simulink model "r2017bSingleARDroneCtrl"  (R2017b)
settings: Solver=FixedStepAuto  StartTime=0.0  StopTime=inf  FixedStep=sampleTime  RelTol=1e-3  EnableMultiTasking=on
values from neighbouring files (symbols this model uses):
  k = 1.0    (= 1)    [start.m]
  k_d_xy = 0.9    [start.m]
  k_d_z = 0.3    [start.m]
  k_l = 5    [start.m]
  k_p_xy = 0.6    [start.m]
  k_p_yaw = 0.5    [start.m]
  k_p_z = 0.6    [start.m]
  k_sign = -1    [start.m]
  limit_cmd_xy = 1    [start.m]
  r_a = 3    [start.m]
  r_M = 2    [start.m]
  r_o = 0.5    [start.m]
  r_s = 0.001    [start.m]
  waypoints = [1,1,1.2,0,0,0,0]'    [start.m]
undefined symbols (not defined in the file or in its folder): Angular, Linear
libraries: robotlib x5
settings Model: Creator=exbot  LastModifiedBy=gzl20
settings DataIOCC: LimitDataPoints=on
settings OptimizationCC: MaxStackSize=64
settings DebuggingCC: ParameterTunabilityLossMsg=error  AllowSymbolicDim=off  SFUnexpectedBacktrackingDiag=warning  SFNoUnconditionalDefaultTransitionDiag=warning  SFExecutionAtInitializationDiag=none
settings HardwareCC: ProdBitPerPointer=32  ProdBitPerSizeT=32  ProdBitPerPtrDiffT=32  ProdLargestAtomicFloat=None  ProdIntDivRoundTo=Undefined  ProdEndianess=Unspecified  ProdWordSize=32  ProdHWDeviceType=Generic->Unspecified (assume 32-bit Generic)
settings ModelReferenceCC: PropagateSignalLabelsOutOfModel=off
settings SFSimCC: MATLABDynamicMemAlloc=off
settings RTWCC: SystemTargetFile=ert.tlc  HardwareBoard=Robot Operating System (ROS)  TemplateMakefile=ert_default_tmf  Toolchain=Catkin  TargetLang=C++
settings CodeAppCC: ForceParamTrailComments=on  IgnoreCustomStorageClasses=off  OperatorAnnotations=on  SimulinkDataObjDesc=on  SFDataObjDesc=on  MATLABFcnDesc=on  InsertBlockDesc=on  StateflowObjectComments=on  MATLABSourceComments=on
settings ERTTargetCC: MultiwordLength=2048  SupportContinuousTime=on
settings ConfigComp: CovMetricSettings=dw  CovHtmlReporting=on  CovSaveCumulativeToWorkspaceVar=on  CovSaveSingleToWorkspaceVar=on  CovExternalEMLEnable=off

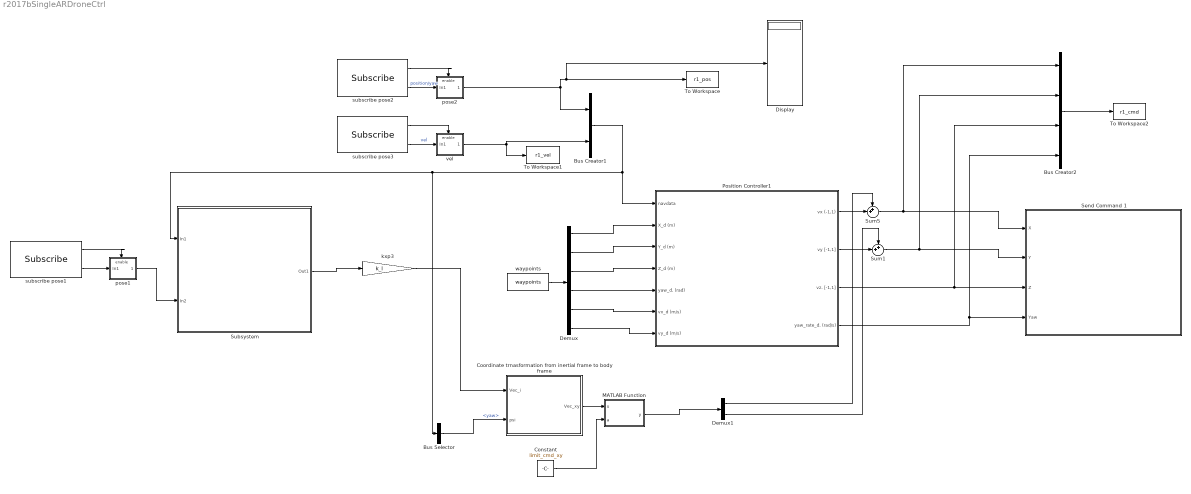
== system r2017bSingleARDroneCtrl ==
  Bus Creator1 : BusCreator  Inputs=2
  Bus Creator2 : BusCreator  Inputs=4
  Bus Selector : BusSelector  OutputSignals=signal1.yaw
  Constant : Constant  Value=limit_cmd_xy
  "Coordinate trnasformation from inertial frame to body frame " : MATLAB Function  TreatAsAtomicUnit=on
  Demux : Demux  Outputs=6
  Demux1 : Demux  Outputs=2
  Display : Display
  MATLAB Function : MATLAB Function  TreatAsAtomicUnit=on
  Position Controller1 : Subsystem  AncestorBlock=ARBlocks/Baseline Controller
  Send Command 1 : Subsystem
  Subsystem : Subsystem
  Sum1 : Sum  Inputs=++|
  Sum5 : Sum  Inputs=++|
  To Workspace : ToWorkspace  VariableName=r1_pos  SaveFormat=Timeseries  SampleTime=-1
  To Workspace1 : ToWorkspace  VariableName=r1_vel  SaveFormat=Timeseries  SampleTime=-1
  To Workspace2 : ToWorkspace  VariableName=r1_cmd  SaveFormat=Timeseries  SampleTime=-1
  kxp3 : Gain  Gain=k_l
  pose1 : Subsystem
  pose2 : Subsystem
  subscribe pose1 : robotlib/Subscribe  SourceLibraryInfo=This block requires Robotics System Toolbox  topicSource=Specify your own  topic=/Obstacle/position  messageType=geometry_msgs/Point  sampleTime=-1  messageQueueLength=1
      settings: SourceProductBaseCode=RO
  subscribe pose2 : robotlib/Subscribe  SourceLibraryInfo=This block requires Robotics System Toolbox  topicSource=Select from ROS network  topic=/Robot_1/pose  messageType=geometry_msgs/PoseStamped  sampleTime=-1  messageQueueLength=1
      settings: SourceProductBaseCode=RO
  subscribe pose3 : robotlib/Subscribe  SourceLibraryInfo=This block requires Robotics System Toolbox  topicSource=Select from ROS network  topic=/Robot_1/vel  messageType=geometry_msgs/PointStamped  sampleTime=-1  messageQueueLength=1
      settings: SourceProductBaseCode=RO
  vel : Subsystem
  waypoints : Constant  Value=waypoints  VectorParams1D=off
  wires:
  Position Controller1/3(vz. [-1,1]) -> Bus Creator2/3, Send Command 1/3(Z)
  Position Controller1/4(yaw_rate_d. (rad/s)) -> Bus Creator2/4, Send Command 1/4(Yaw)
  Bus Creator2/1 -> To Workspace2/1
  pose2/1(Out1) -> Bus Creator1/1, Display/1, To Workspace/1
  vel/1(Out1) -> Bus Creator1/2, To Workspace1/1
  Bus Creator1/1 -> Bus Selector/1, Subsystem/1(In1), Position Controller1/1(navdata)
  subscribe pose2/2 -> pose2/1(In1)  "position/yaw"
  subscribe pose2/1 -> pose2/Enable
  subscribe pose3/2 -> vel/1(In1)  "vel"
  subscribe pose3/1 -> vel/Enable
  subscribe pose1/2 -> pose1/1(In1)
  subscribe pose1/1 -> pose1/Enable
  pose1/1(Out1) -> Subsystem/2(In2)
  Subsystem/1(Out1) -> kxp3/1
  waypoints/1 -> Demux/1
  Demux/1 -> Position Controller1/2(X_d (m))
  Demux/2 -> Position Controller1/3(Y_d (m))
  Demux/3 -> Position Controller1/4(Z_d (m))
  Demux/4 -> Position Controller1/5(yaw_d. (rad))
  Demux/5 -> Position Controller1/6(vx_d (m/s))
  Demux/6 -> Position Controller1/7(vy_d (m/s))
  kxp3/1 -> "Coordinate trnasformation from inertial frame to body frame "/1(Vec_i)
  Position Controller1/1(vx (-1,1)) -> Sum5/2
  Sum5/1 -> Bus Creator2/1, Send Command 1/1(X)
  Sum1/1 -> Bus Creator2/2, Send Command 1/2(Y)
  Position Controller1/2(vy [-1,1]) -> Sum1/2
  Constant/1 -> MATLAB Function/2(a)
  "Coordinate trnasformation from inertial frame to body frame "/1(Vec_xy) -> MATLAB Function/1(u)
  Bus Selector/1 -> "Coordinate trnasformation from inertial frame to body frame "/2(psi)  "<yaw>"
  MATLAB Function/1(y) -> Demux1/1
  Demux1/1 -> Sum5/1
  Demux1/2 -> Sum1/1

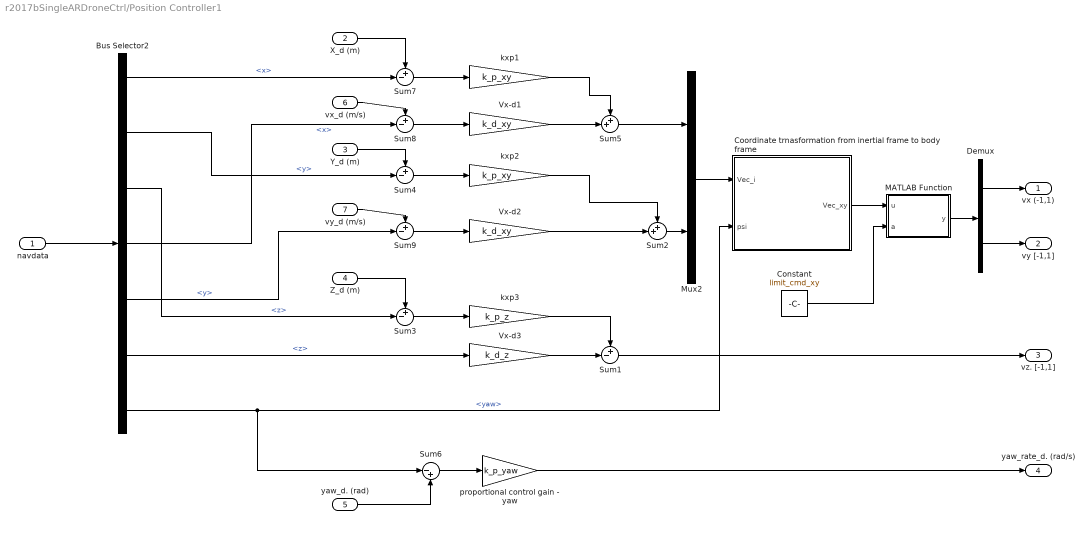
== system r2017bSingleARDroneCtrl/Position Controller1 ==
  navdata : Inport
  X_d (m) : Inport  Port=2
  Y_d (m) : Inport  Port=3
  Z_d (m) : Inport  Port=4
  yaw_d. (rad) : Inport  Port=5
  vx_d (m/s) : Inport  Port=6
  vy_d (m/s) : Inport  Port=7
  Bus Selector2 : BusSelector  OutputSignals=signal1.x,signal1.y,signal1.z,signal2.x,signal2.y,signal2.z,signal1.yaw
  Constant : Constant  Value=limit_cmd_xy
  "Coordinate trnasformation from inertial frame to body frame " : MATLAB Function  TreatAsAtomicUnit=on
  Demux : Demux  Outputs=2
  MATLAB Function : MATLAB Function  TreatAsAtomicUnit=on
  Mux2 : Mux  Inputs=2
  Sum{1,3..4,7..9} (6 alike) : Sum  Inputs=+-|
  Sum2 : Sum  Inputs=++|
  Sum5 : Sum  Inputs=++|
  Sum6 : Sum  Inputs=|-+
  Vx-d1 : Gain  Gain=k_d_xy
  Vx-d2 : Gain  Gain=k_d_xy
  Vx-d3 : Gain  Gain=k_d_z
  kxp1 : Gain  Gain=k_p_xy
  kxp2 : Gain  Gain=k_p_xy
  kxp3 : Gain  Gain=k_p_z
  proportional control gain - yaw : Gain  Gain=k_p_yaw
  vx (-1,1) : Outport
  vy [-1,1] : Outport  Port=2
  vz. [-1,1] : Outport  Port=3
  yaw_rate_d. (rad/s) : Outport  Port=4
  wires:
  MATLAB Function/1(y) -> Demux/1
  Demux/1 -> vx (-1,1)/1
  Demux/2 -> vy [-1,1]/1
  Constant/1 -> MATLAB Function/2(a)
  Mux2/1 -> "Coordinate trnasformation from inertial frame to body frame "/1(Vec_i)
  Sum7/1 -> kxp1/1
  kxp1/1 -> Sum5/1
  Vx-d1/1 -> Sum5/2
  X_d (m)/1 -> Sum7/1
  Sum4/1 -> kxp2/1
  kxp2/1 -> Sum2/1
  Vx-d2/1 -> Sum2/2
  Y_d (m)/1 -> Sum4/1
  Sum3/1 -> kxp3/1
  kxp3/1 -> Sum1/1
  Vx-d3/1 -> Sum1/2
  Z_d (m)/1 -> Sum3/1
  Bus Selector2/1 -> Sum7/2  "<x>"
  Bus Selector2/2 -> Sum4/2  "<y>"
  Bus Selector2/3 -> Sum3/2  "<z>"
  Bus Selector2/6 -> Vx-d3/1  "<z>"
  Bus Selector2/7 -> Sum6/1, "Coordinate trnasformation from inertial frame to body frame "/2(psi)  "<yaw>"
  Sum6/1 -> proportional control gain - yaw/1
  proportional control gain - yaw/1 -> yaw_rate_d. (rad/s)/1
  yaw_d. (rad)/1 -> Sum6/2
  navdata/1 -> Bus Selector2/1
  Sum5/1 -> Mux2/1
  Sum2/1 -> Mux2/2
  Sum1/1 -> vz. [-1,1]/1
  "Coordinate trnasformation from inertial frame to body frame "/1(Vec_xy) -> MATLAB Function/1(u)
  Bus Selector2/4 -> Sum8/2  "<x>"
  vx_d (m/s)/1 -> Sum8/1
  Sum8/1 -> Vx-d1/1
  Sum9/1 -> Vx-d2/1
  Bus Selector2/5 -> Sum9/2  "<y>"
  vy_d (m/s)/1 -> Sum9/1

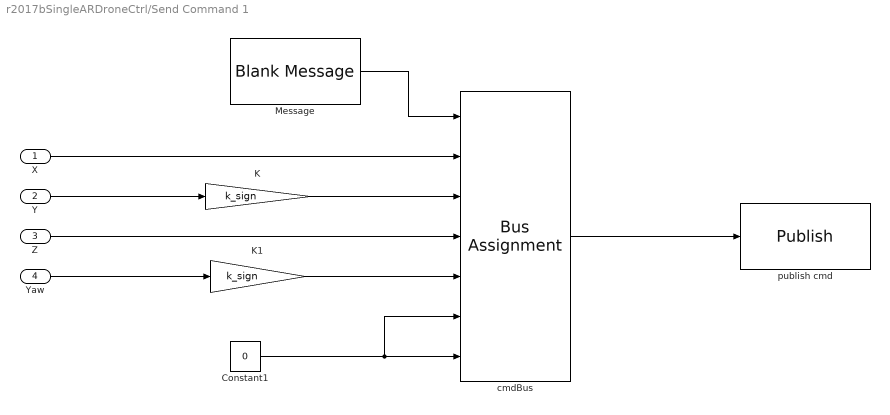
== system r2017bSingleARDroneCtrl/Send Command 1 ==
  X : Inport
  Y : Inport  Port=2
  Z : Inport  Port=3
  Yaw : Inport  Port=4
  " Message" : robotlib/Blank Message  SourceLibraryInfo=This block requires Robotics System Toolbox  messageType=geometry_msgs/Twist  SampleTime=inf
      settings: SourceProductBaseCode=RO
  Constant1 : Constant  Value=0
  K : Gain  Gain=k_sign
  K1 : Gain  Gain=k_sign
  cmdBus : BusAssignment  AssignedSignals=Linear.X,Linear.Y,Linear.Z,Angular.Z,Angular.X,Angular.Y
  publish cmd : robotlib/Publish  SourceLibraryInfo=This block requires Robotics System Toolbox  topicSource=Select from ROS network  topic=/bebop1/cmd_vel  messageType=geometry_msgs/Twist  messageQueueLength=1
      settings: SourceProductBaseCode=RO
  wires:
  cmdBus/1 -> publish cmd/1
  Constant1/1 -> cmdBus/6, cmdBus/7
  K/1 -> cmdBus/3
  K1/1 -> cmdBus/5
  " Message"/1 -> cmdBus/1
  X/1 -> cmdBus/2
  Y/1 -> K/1
  Z/1 -> cmdBus/4
  Yaw/1 -> K1/1

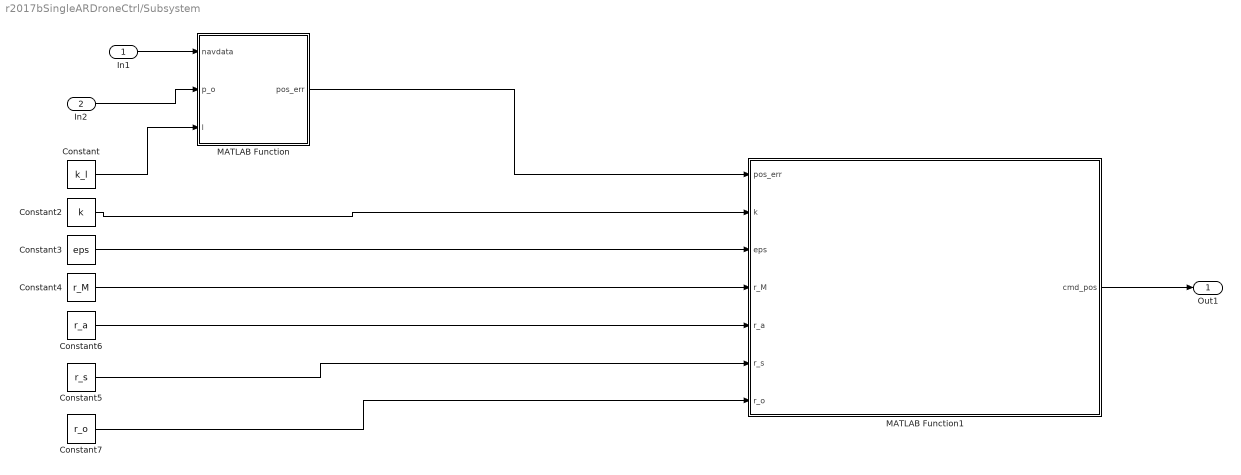
== system r2017bSingleARDroneCtrl/Subsystem ==
  In1 : Inport
  In2 : Inport  Port=2
  Constant : Constant  Value=k_l
  Constant2 : Constant  Value=k
  Constant3 : Constant  Value=eps
  Constant4 : Constant  Value=r_M
  Constant5 : Constant  Value=r_s
  Constant6 : Constant  Value=r_a
  Constant7 : Constant  Value=r_o
  MATLAB Function : MATLAB Function  TreatAsAtomicUnit=on
  MATLAB Function1 : MATLAB Function  TreatAsAtomicUnit=on
  Out1 : Outport
  wires:
  In1/1 -> MATLAB Function/1(navdata)
  In2/1 -> MATLAB Function/2(p_o)
  MATLAB Function/1(pos_err) -> MATLAB Function1/1(pos_err)
  Constant/1 -> MATLAB Function/3(l)
  Constant2/1 -> MATLAB Function1/2(k)
  Constant3/1 -> MATLAB Function1/3(eps)
  Constant4/1 -> MATLAB Function1/4(r_M)
  Constant6/1 -> MATLAB Function1/5(r_a)
  Constant5/1 -> MATLAB Function1/6(r_s)
  Constant7/1 -> MATLAB Function1/7(r_o)
  MATLAB Function1/1(cmd_pos) -> Out1/1

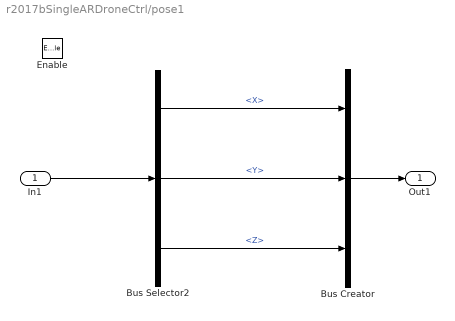
== system r2017bSingleARDroneCtrl/pose1 ==
  In1 : Inport
  Enable : EnablePort
  Bus Creator : BusCreator  Inputs=3
  Bus Selector2 : BusSelector  OutputSignals=X,Y,Z
  Out1 : Outport
  wires:
  Bus Creator/1 -> Out1/1
  In1/1 -> Bus Selector2/1
  Bus Selector2/1 -> Bus Creator/1  "<X>"
  Bus Selector2/2 -> Bus Creator/2  "<Y>"
  Bus Selector2/3 -> Bus Creator/3  "<Z>"

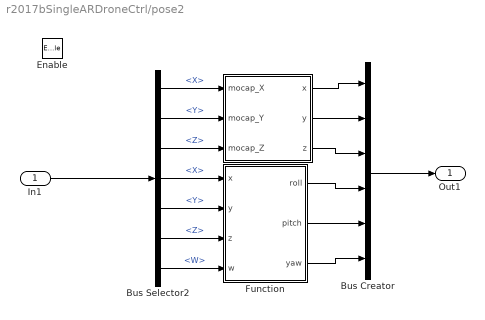
== system r2017bSingleARDroneCtrl/pose2 ==
  In1 : Inport
  Enable : EnablePort
  " " : MATLAB Function  TreatAsAtomicUnit=on
  " Function" : MATLAB Function  TreatAsAtomicUnit=on
  Bus Creator : BusCreator  Inputs=6
  Bus Selector2 : BusSelector  OutputSignals=Pose.Position.X,Pose.Position.Y,Pose.Position.Z,Pose.Orientation.X,Pose.Orientation.Y,Pose.Orientation.Z,Pose.Orientation.W
  Out1 : Outport
  wires:
  Bus Creator/1 -> Out1/1
  In1/1 -> Bus Selector2/1
  " Function"/1(roll) -> Bus Creator/4
  " Function"/2(pitch) -> Bus Creator/5
  " Function"/3(yaw) -> Bus Creator/6
  Bus Selector2/4 -> " Function"/1(x)  "<X>"
  Bus Selector2/5 -> " Function"/2(y)  "<Y>"
  Bus Selector2/6 -> " Function"/3(z)  "<Z>"
  Bus Selector2/7 -> " Function"/4(w)  "<W>"
  Bus Selector2/1 -> " "/1(mocap_X)  "<X>"
  Bus Selector2/2 -> " "/2(mocap_Y)  "<Y>"
  Bus Selector2/3 -> " "/3(mocap_Z)  "<Z>"
  " "/1(x) -> Bus Creator/1
  " "/2(y) -> Bus Creator/2
  " "/3(z) -> Bus Creator/3

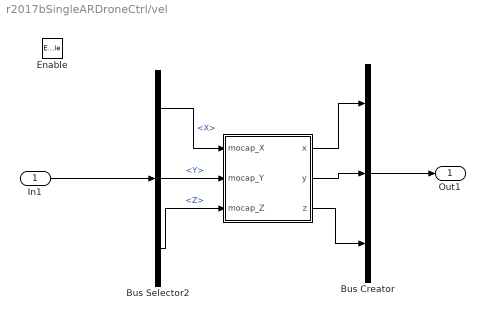
== system r2017bSingleARDroneCtrl/vel ==
  In1 : Inport
  Enable : EnablePort
  " " : MATLAB Function  TreatAsAtomicUnit=on
  Bus Creator : BusCreator  Inputs=3
  Bus Selector2 : BusSelector  OutputSignals=Point.X,Point.Y,Point.Z
  Out1 : Outport
  wires:
  Bus Creator/1 -> Out1/1
  In1/1 -> Bus Selector2/1
  Bus Selector2/1 -> " "/1(mocap_X)  "<X>"
  Bus Selector2/2 -> " "/2(mocap_Y)  "<Y>"
  Bus Selector2/3 -> " "/3(mocap_Z)  "<Z>"
  " "/1(x) -> Bus Creator/1
  " "/2(y) -> Bus Creator/2
  " "/3(z) -> Bus Creator/3

== matlab function r2017bSingleARDroneCtrl/Subsystem/MATLAB Function1 ==
  data: pos_err input; cmd_pos output; k input; eps input; r_M input; r_a input; r_s input; r_o input
function cmd_pos=V_o(pos_err,k,eps,r_M,r_a,r_s,r_o)
    t=norm(pos_err);
    r_Mo = r_M+r_o;
    r_ao = r_a+r_o;
    f = k*sig(t,r_Mo,r_ao);
    f_grad = k*grad_sig(t,r_Mo,r_ao);
    g = (1 +eps) * t - r_Mo * s_m(t/r_Mo, r_s);
    g_grad = (1 + eps) - grad_s_m(t/r_Mo, r_s);
    V = (f_grad*g-f*g_grad)/(g*g);
    cmd_pos = V*(pos_err)/t;
end

function sig_out=sig(x,  d1, d2)
     A = -2/((d1-d2)*(d1-d2)*(d1-d2));
     B =  3*(d1+d2)/((d1-d2)*(d1-d2)*(d1-d2));
     C = -6*d1*d2/((d1-d2)*(d1-d2)*(d1-d2));
     D = d2*d2*(3*d1-d2)/((d1-d2)*(d1-d2)*(d1-d2));

    if (x<d1)
        sig_out = 1.0;
    elseif (x>d2)
        sig_out= 0.0;
    else
        sig_out= A*x*x*x+B*x*x+C*x+D;
    end
end

function grad_sig_out=grad_sig( x,  d1, d2)

    A = -2/((d1-d2)*(d1-d2)*(d1-d2));
    B =  3*(d1+d2)/((d1-d2)*(d1-d2)*(d1-d2));
    C = -6*d1*d2/((d1-d2)*(d1-d2)*(d1-d2));
    D = d2*d2*(3*d1-d2)/((d1-d2)*(d1-d2)*(d1-d2));

    if (x<d1)
        grad_sig_out = 1.0;
    elseif (x>d2)
        grad_sig_out= 0.0;
    else
        grad_sig_out=  3*A*x*x+2*B*x+C;
    end
end

function s_m_out=s_m(x, rs)

    x2 = 1+rs*(1/tan(67.5/180*pi));
    x1 = x2 - rs*sin(45/180*pi);

    if (x>=0 && x<x1)
        s_m_out = x;
    elseif (x >x2)
        s_m_out= 1.0;
    else
        s_m_out = (1-rs)+sqrt(rs*rs-(x-x2)*(x-x2));
    end
end

function grad_s_m_out=grad_s_m(x, rs)
    x2 = 1+rs*(1/tan(67.5/180*pi));
    x1 = x2 - rs*sin(45/180*pi);

    if (x>=0 && x<x1)
        grad_s_m_out = 1.0;
    elseif (x >x2)
        grad_s_m_out = 0.0;
    else
        grad_s_m_out= (x2-x)/sqrt(rs*rs-(x-x2)*(x-x2));
    end
end

== matlab function r2017bSingleARDroneCtrl/Subsystem/MATLAB Function ==
  data: navdata input; pos_err output; p_o input; l input
function pos_err = fcn(navdata, p_o,l) % navdata: x y z yaw vx vy vz
x_err =p_o(1)-navdata(1)+1/l*navdata(5); % po_x-px+1/l*vx
y_err =p_o(2)-navdata(2)+1/l*navdata(6);
pos_err = [x_err,y_err]';

== matlab function r2017bSingleARDroneCtrl/Coordinate trnasformation from inertial frame to body frame  ==
  data: Vec_i input; Vec_xy output; psi input
function Vec_xy  = fcn(Vec_i , psi)
%#codegen
T = [cos(psi) sin(psi) ; -sin(psi) cos(psi)] ; 
Vec_xy = T*Vec_i(1:2,1);

== matlab function r2017bSingleARDroneCtrl/MATLAB Function ==
  data: u input; y output; a input
function y = fcn(u,a)
    temp = norm(u,Inf);
    if  temp<=a
        y = u;
    else
        y= a*u/temp;
    end
end

== matlab function r2017bSingleARDroneCtrl/Position Controller1/MATLAB Function ==
  data: u input; y output; a input
function y = fcn(u,a)
    temp = norm(u,Inf);
    if  temp<=a
        y = u;
    else
        y= a*u/temp;
    end
end

== matlab function r2017bSingleARDroneCtrl/pose2/  ==
  data: x output; mocap_X input; y output; mocap_Y input; mocap_Z input; z output
function [x, y, z] = xyz_tf(mocap_X, mocap_Y, mocap_Z)
x =  -mocap_Y;
y =  -mocap_X;
z =  mocap_Z;

== matlab function r2017bSingleARDroneCtrl/pose2/ Function ==
  data: x input; roll output; y input; z input; w input; pitch output; yaw output
function [roll, pitch, yaw] = quat2rpy(x, y, z, w)
    t0 = -2.0 * (y * y + z * z) + 1.0;
    t1 = +2.0 * (x * y + w * z);
    t2 = -2.0 * (x * z - w * y);
    t3 = +2.0 * (y * z + w * x);
    t4 = -2.0 * (x * x + y * y) + 1.0;

    roll = -asin(t2);
    pitch = -atan2(t3, t4);
    yaw= -atan2(t1, t0);

== matlab function r2017bSingleARDroneCtrl/vel/  ==
  data: x output; mocap_X input; y output; mocap_Y input; mocap_Z input; z output
function [x, y, z] = xyz_tf(mocap_X, mocap_Y, mocap_Z)
x = - mocap_Y;
y = - mocap_X;
z = mocap_Z;

== matlab function r2017bSingleARDroneCtrl/Position Controller1/Coordinate trnasformation from inertial frame to body frame  ==
  data: Vec_i input; Vec_xy output; psi input
function Vec_xy  = fcn(Vec_i , psi)
%#codegen
T = [cos(psi) sin(psi) ; -sin(psi) cos(psi)] ; 
Vec_xy = T*Vec_i(1:2,1);
